simulink model "Sim_control_FC"  (R2021a)
settings: Solver=VariableStepAuto  StartTime=0.0  StopTime=simulation_time  RelTol=1e-3
values from neighbouring files (symbols this model uses):
  K_d = 0    [test_script (1).m]    (also in test_script.m)
  K_i = 0    [test_script (1).m]    (also in test_script.m)
  K_p = 10    [test_script (1).m]    (also in test_script.m)
  n_cells = 40    [test_script (1).m]    (also in test_script.m)
  step_time = 1    [test_script (1).m]    (also in test_script.m)
libraries: pid_lib x1
settings Model: Creator=JM  LastModifiedBy=simao
settings SolverCC: AlgebraicLoopSolver=TrustRegion
settings DebuggingCC: SFMachineParentedDataDiag=warning

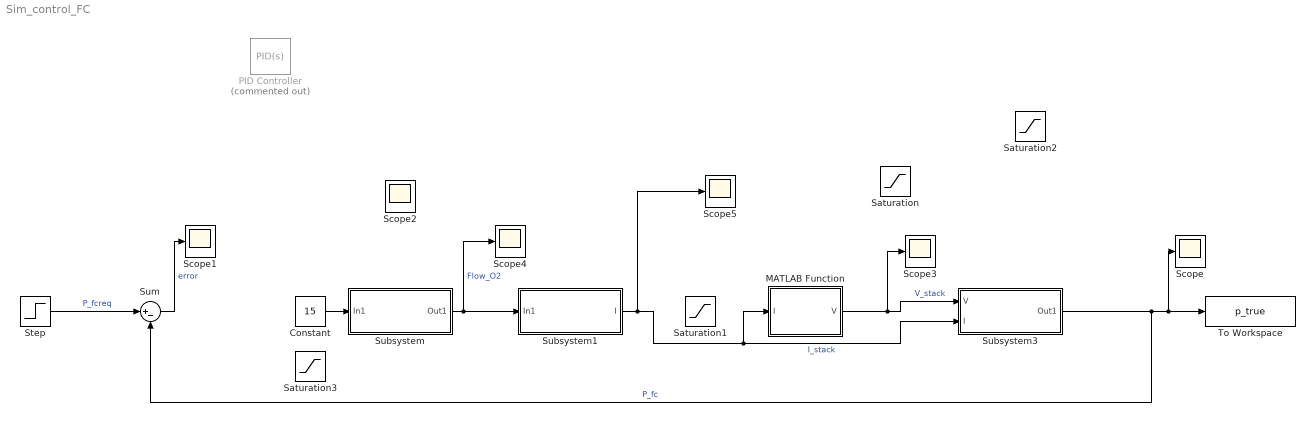
== system Sim_control_FC ==
  Constant : Constant  Value=15
  MATLAB Function : MATLAB Function  TreatAsAtomicUnit=on
  PID Controller : pid_lib/PID Controller  Commented=on  Controller=PID  Form=Parallel  TimeDomain=Continuous-time  UseExternalTs=off  SampleTime=-1  IntegratorMethod=Forward Euler  FilterMethod=Forward Euler  ControllerParametersSource=internal  P=K_p  I=K_i  D=K_d  UseFilter=on  N=100  TunerSelectOption=Transfer Function Based (PID Tuner App)  InitialConditionSource=internal  InitialConditionForIntegrator=15  InitialConditionForFilter=0  DifferentiatorICPrevScaledInput=0  ExternalReset=none  TrackingMode=off  Kt=1  LimitOutput=off  SatLimitsSource=internal  UpperSaturationLimit=inf  LowerSaturationLimit=-inf  LinearizeAsGain=on  AntiWindupMode=none  Kb=1  POutMin=[]  POutMax=[]  IOutMin=[]  IOutMax=[]  DOutMin=[]  DOutMax=[]  NOutMin=[]  NOutMax=[]  SumOutMin=[]  SumOutMax=[]  SaturationOutMin=[]  SaturationOutMax=[]  PParamMin=[]  PParamMax=[]  IParamMin=[]  IParamMax=[]  DParamMin=[]  DParamMax=[]  NParamMin=[]  NParamMax=[]  KbParamMin=[]  KbParamMax=[]  KtParamMin=[]  KtParamMax=[]  KbOutMin=[]  KbOutMax=[]  KtOutMin=[]  KtOutMax=[]  IntegratorOutMin=[]  IntegratorOutMax=[]  FilterOutMin=[]  FilterOutMax=[]  SumI1OutMin=[]  SumI1OutMax=[]  SumI2OutMin=[]  SumI2OutMax=[]  SumI3OutMin=[]  SumI3OutMax=[]  SumI4OutMin=[]  SumI4OutMax=[]  SumDOutMin=[]  SumDOutMax=[]  DifferentiatorOutMin=[]  DifferentiatorOutMax=[]  FilterDiffOutCoefMin=[]  FilterDiffOutCoefMax=[]  ReciprocalOutMin=[]  ReciprocalOutMax=[]  SumDenOutMin=[]  SumDenOutMax=[]  SumNumOutMin=[]  SumNumOutMax=[]  DivideOutMin=[]  DivideOutMax=[]  UdiffTsProdOutMin=[]  UdiffTsProdOutMax=[]  NTsProdOutMin=[]  NTsProdOutMax=[]  UintegralTsProdOutMin=[]  UintegralTsProdOutMax=[]  UngainTsProdOutMin=[]  UngainTsProdOutMax=[]  IntegratorContinuousStateAttributes=''  IntegratorStateMustResolveToSignalObject=off  IntegratorRTWStateStorageClass=Auto  FilterContinuousStateAttributes=''  FilterStateMustResolveToSignalObject=off  FilterRTWStateStorageClass=Auto  ParallelPVariant=InternalParameters  IdealPVariant=Disabled  IVariant=InternalParameters  DVariant=InternalParameters  IntegratorVariant=Continuous  SatVariant=Disabled  AWVariant=Passthrough  PCopyVariant=Disabled  TRVariant=Disabled  FdbkBlocksVariant=Forward  IdealPFdbkVariant=Disabled  SatFdbkVariant=Disabled  DerivativeFilterVariant=ContFilter  NVariant=InternalParameters  NCopyVariant=Disabled  FilterICVariant=InternalICsFilter  IntegratorICVariant=InternalICs  ExternalResetVariant=Disabled  TRSumVariant=Passthrough  SumFdbkVariant=Disabled  SumVariant=Sum_PID  TsampFilterVariant=InternalTs  TsampNgainVariant=Passthrough  TsampIntegralVariant=Passthrough  ExternalSaturationOutDataTypeStr=Inherit: Same as second input
  Saturation : Saturate  UpperLimit=41  LowerLimit=9
  Saturation1 : Saturate  UpperLimit=230  LowerLimit=0
  Saturation2 : Saturate  UpperLimit=10000  LowerLimit=0
  Saturation3 : Saturate  UpperLimit=24  LowerLimit=15
  Scope{,1..5} (6 alike) : Scope
  Step : Step  Time=step_time  SampleTime=0
  Subsystem : Subsystem
  Subsystem1 : Subsystem
  Subsystem3 : Subsystem
  Sum : Sum  Inputs=|+-
  To Workspace : ToWorkspace  VariableName=p_true  SaveFormat=Structure With Time  SampleTime=-1
  wires:
  Sum/1 -> Scope1/1  "error"
  Step/1 -> Sum/1  "P_fcreq"
  Subsystem/1(Out1) -> Scope4/1, Subsystem1/1(In1)  "Flow_O2"
  Subsystem3/1(Out1) -> Scope/1, To Workspace/1, Sum/2  "P_fc"
  Subsystem1/1(I) -> Scope5/1, Subsystem3/2(I), MATLAB Function/1(I)  "I_stack"
  MATLAB Function/1(V) -> Scope3/1, Subsystem3/1(V)  "V_stack"
  Constant/1 -> Subsystem/1(In1)

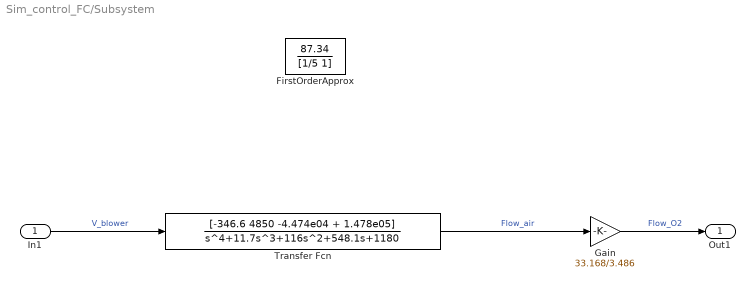
== system Sim_control_FC/Subsystem ==
  In1 : Inport
  FirstOrderApprox : TransferFcn  Numerator=[87.34]  Denominator=[1/5 1]
  Gain : Gain  Gain=33.168/3.486
  Transfer Fcn : TransferFcn  Numerator=[-346.6 4850 -4.474e04 + 1.478e05]  Denominator=[1 11.7 116 548.1 1180]
  Out1 : Outport
  wires:
  Gain/1 -> Out1/1  "Flow_O2"
  In1/1 -> Transfer Fcn/1  "V_blower"
  Transfer Fcn/1 -> Gain/1  "Flow_air"

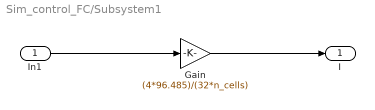
== system Sim_control_FC/Subsystem1 ==
  In1 : Inport
  Gain : Gain  Gain=(4*96.485)/(32*n_cells)
  I : Outport
  wires:
  In1/1 -> Gain/1
  Gain/1 -> I/1

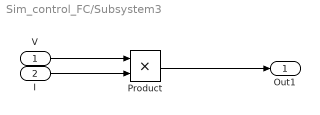
== system Sim_control_FC/Subsystem3 ==
  V : Inport
  I : Inport  Port=2
  Product : Product
  Out1 : Outport
  wires:
  I/1 -> Product/2
  V/1 -> Product/1
  Product/1 -> Out1/1

== matlab function Sim_control_FC/MATLAB Function ==
  data: I input; V output
function V = Stack_voltage(I)
I_stack = [0 10 40 80 120 150 180 200 230];
V_stack = [38.7 34.3 31.6 29.3 27.5 26.2 24.8 23.8 22.1];

%I = linspace(max (I_stack), min(I_stack), 500);
V = interp1(I_stack, V_stack, I, 'linear');
